simulink model "ode_3state"  (Simulink 7.8)
settings: Solver=ode4  StartTime=0.0  StopTime=time_span  RelTol=1e-3
values from neighbouring files (symbols this model uses):
  IC = p.simulation.IC    [RunModel.m]    (also in RunModel3.m = ICs(i,:); RunModel4.m = ICs(i,:); RunTargetModel.m)
  outstr1 = models{1}    [RunModel3.m]    (also in RunModel4.m)
  outstr2 = models{2}    [RunModel3.m]    (also in RunModel4.m)
  outstr3 = models{3}    [RunModel3.m]    (also in RunModel4.m)
  samp_time = p.simulation.samp_time    [RunCtrlModel.m]    (also in RunCtrlModel_sym.m; RunModel.m = time_span/(p.simulation.ndata-1); RunModel3.m = time_span/(p.simulation.ndata-1); RunModel4.m = time_span/(p.simulation.ndata-1))
settings Model: Creator=Kourosh Danai  LastModifiedBy=WECava
settings DataIOCC: SaveFormat=StructureWithTime  TimeSaveName=t  OutputSaveName=y
settings DebuggingCC: AlgebraicLoopMsg=none  FcnCallInpInsideContextMsg=Use local settings  StrictBusMsg=Warning
settings SFSimCC: SimParseCustomCode=off

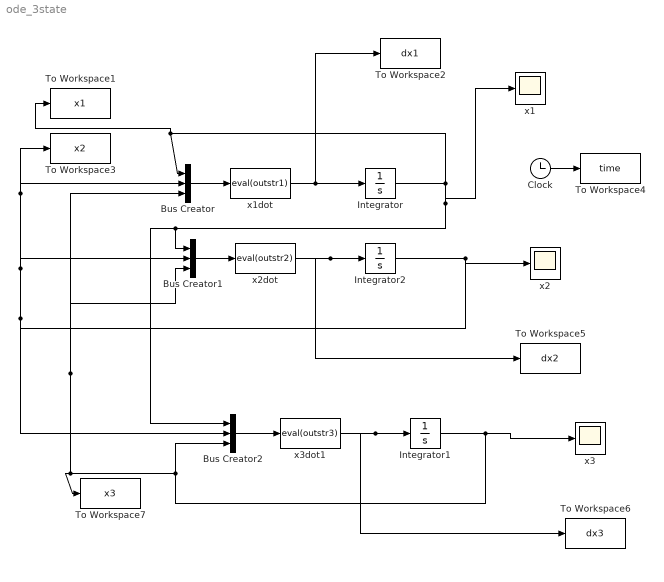
== system ode_3state ==
  Bus Creator : BusCreator  Inputs=3
  Bus Creator1 : BusCreator  Inputs=3
  Bus Creator2 : BusCreator  Inputs=3
  Clock : Clock
  Integrator : Integrator  InitialCondition=IC(1)
  Integrator1 : Integrator  InitialCondition=IC(3)
  Integrator2 : Integrator  InitialCondition=IC(2)
  To Workspace1 : ToWorkspace  VariableName=x1  SampleTime=-1  SaveFormat=Array
  To Workspace2 : ToWorkspace  VariableName=dx1  SampleTime=-1  SaveFormat=Array
  To Workspace3 : ToWorkspace  VariableName=x2  SampleTime=-1  SaveFormat=Array
  To Workspace4 : ToWorkspace  VariableName=time  SampleTime=-1  SaveFormat=Array
  To Workspace5 : ToWorkspace  VariableName=dx2  SampleTime=-1  SaveFormat=Array
  To Workspace6 : ToWorkspace  VariableName=dx3  SampleTime=-1  SaveFormat=Array
  To Workspace7 : ToWorkspace  VariableName=x3  SampleTime=-1  SaveFormat=Array
  x1 : Scope
  x1dot : MATLABFcn  MATLABFcn=eval(outstr1)  SampleTime=samp_time
  x2 : Scope
      settings: SaveName=ScopeData2
  x2dot : MATLABFcn  MATLABFcn=eval(outstr2)
  x3 : Scope
  x3dot1 : MATLABFcn  MATLABFcn=eval(outstr3)
  wires:
  Bus Creator/1 -> x1dot/1
  Bus Creator1/1 -> x2dot/1
  Integrator/1 -> x1/1, Bus Creator1/1, Bus Creator2/1, Bus Creator/1, To Workspace1/1
  Integrator2/1 -> x2/1, Bus Creator/2, To Workspace3/1, Bus Creator1/2, Bus Creator2/2
  x1dot/1 -> Integrator/1, To Workspace2/1
  x2dot/1 -> Integrator2/1, To Workspace5/1
  Bus Creator2/1 -> x3dot1/1
  Integrator1/1 -> x3/1, Bus Creator2/3, Bus Creator1/3, Bus Creator/3, To Workspace7/1
  x3dot1/1 -> Integrator1/1, To Workspace6/1
  Clock/1 -> To Workspace4/1
